simulink model "tilstandsmodelReducedOBS"  (Simulink 7.4)
settings: Solver=ode45  StartTime=0.0  StopTime=200  FixedStep=0.001  RelTol=1e-3
values from neighbouring files (symbols this model uses):
  A = [((-(Km^2)/(Rm*Jt))-(bs/Jt)) 0 0 0 ... (first row only)    [tilstandsREG.m]
  Aro = [0 ((3*g)/(lp*2));1 0]    [tilstandsREG.m]
  B = [1.292*(Km/(Jt*Rm)) ... (first row only)    [tilstandsREG.m]
  Bro = [1;0]    [tilstandsREG.m]
  C = [1 0 0 0 ... (first row only)    [tilstandsREG.m]
  Cro = [0 -(9*la*g)/(4*lp^2)]    [tilstandsREG.m]
  Dro = [-(3*la)/(2*lp)]    [tilstandsREG.m]
  F = Fe(:,1:4)    [tilstandsREG.m]
  Fi = Fe(:,5)    [tilstandsREG.m]
  Km = 0.022141706562986    (= 0.022141706563)    [pindregStart.m]    (also in tilstandsREG.m)
  Lro = (-place(Aro',Cro',[-35;-36]))'    [tilstandsREG.m]
  Rm = 0.807790757873553    (= 0.807790757874)    [pindregStart.m]    (also in tilstandsREG.m)
libraries: vrlib x3, simulink x1
settings Model: Creator=Skov  LastModifiedBy=Skov

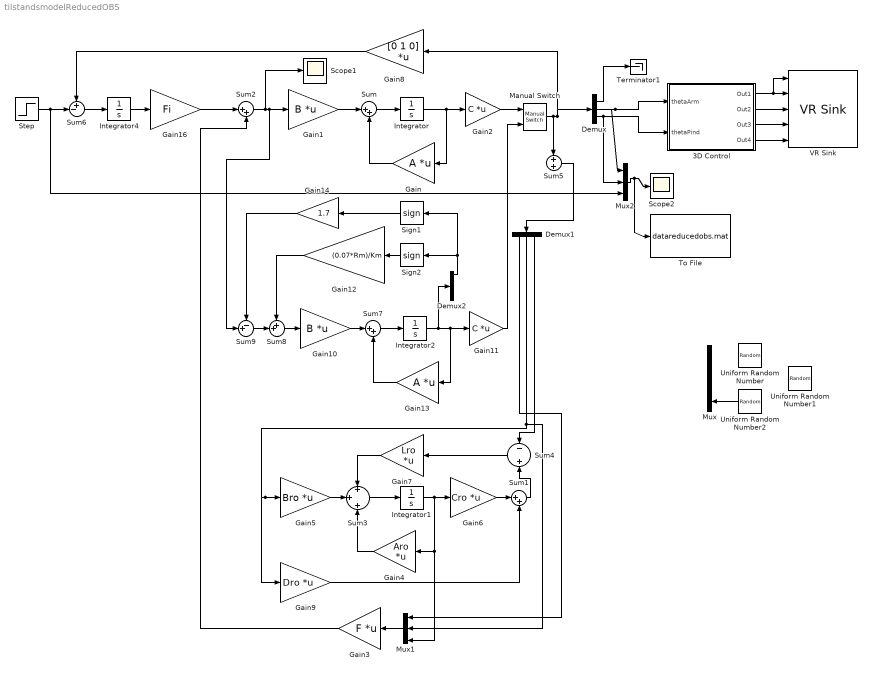
== system tilstandsmodelReducedOBS ==
  3D Control : Subsystem
  Demux : Demux  Outputs=3
  Demux1 : Demux  Outputs=3
  Demux2 : Demux
  Gain : Gain  Gain=A  Multiplication=Matrix(K*u)  ParameterDataType=fixdt(1, 16)  ParameterScaling=2^0  OutDataType=fixdt(1, 16)  OutScaling=2^0
  Gain1 : Gain  Gain=B  Multiplication=Matrix(K*u)  ParameterDataType=fixdt(1, 16)  ParameterScaling=2^0  OutDataType=fixdt(1, 16)  OutScaling=2^0
  Gain10 : Gain  Gain=B  Multiplication=Matrix(K*u)  ParameterDataType=fixdt(1, 16)  ParameterScaling=2^0  OutDataType=fixdt(1, 16)  OutScaling=2^0
  Gain11 : Gain  Gain=C  Multiplication=Matrix(K*u)  ParameterDataType=fixdt(1, 16)  ParameterScaling=2^0  OutDataType=fixdt(1, 16)  OutScaling=2^0
  Gain12 : Gain  Gain=(0.07*Rm)/Km  ParameterDataType=fixdt(1, 16)  ParameterScaling=2^0  OutDataType=fixdt(1, 16)  OutScaling=2^0
  Gain13 : Gain  Gain=A  Multiplication=Matrix(K*u)  ParameterDataType=fixdt(1, 16)  ParameterScaling=2^0  OutDataType=fixdt(1, 16)  OutScaling=2^0
  Gain14 : Gain  Gain=1.7  ParameterDataType=fixdt(1, 16)  ParameterScaling=2^0  OutDataType=fixdt(1, 16)  OutScaling=2^0
  Gain16 : Gain  Gain=Fi  ParameterDataType=fixdt(1, 16)  ParameterScaling=2^0  OutDataType=fixdt(1, 16)  OutScaling=2^0
  Gain2 : Gain  Gain=C  Multiplication=Matrix(K*u)  ParameterDataType=fixdt(1, 16)  ParameterScaling=2^0  OutDataType=fixdt(1, 16)  OutScaling=2^0
  Gain3 : Gain  Gain=F  Multiplication=Matrix(K*u)  ParameterDataType=fixdt(1, 16)  ParameterScaling=2^0  OutDataType=fixdt(1, 16)  OutScaling=2^0
  Gain4 : Gain  Gain=Aro  Multiplication=Matrix(K*u)  ParameterDataType=fixdt(1, 16)  ParameterScaling=2^0  OutDataType=fixdt(1, 16)  OutScaling=2^0
  Gain5 : Gain  Gain=Bro  Multiplication=Matrix(K*u)  ParameterDataType=fixdt(1, 16)  ParameterScaling=2^0  OutDataType=fixdt(1, 16)  OutScaling=2^0
  Gain6 : Gain  Gain=Cro  Multiplication=Matrix(K*u)  ParameterDataType=fixdt(1, 16)  ParameterScaling=2^0  OutDataType=fixdt(1, 16)  OutScaling=2^0
  Gain7 : Gain  Gain=Lro  Multiplication=Matrix(K*u)  ParameterDataType=fixdt(1, 16)  ParameterScaling=2^0  OutDataType=fixdt(1, 16)  OutScaling=2^0
  Gain8 : Gain  Gain=[0 1 0]  Multiplication=Matrix(K*u)  ParameterDataType=fixdt(1, 16)  ParameterScaling=2^0  OutDataType=fixdt(1, 16)  OutScaling=2^0
  Gain9 : Gain  Gain=Dro  Multiplication=Matrix(K*u)  ParameterDataType=fixdt(1, 16)  ParameterScaling=2^0  OutDataType=fixdt(1, 16)  OutScaling=2^0
  Integrator : Integrator  InitialCondition=[0 0 0 0]
  Integrator1 : Integrator  InitialCondition=[0 0]
  Integrator2 : Integrator  InitialCondition=[0 0 0 0]
  Integrator4 : Integrator  InitialCondition=[0]
  Manual Switch : simulink/Signal Routing/Manual Switch  SystemSampleTime=-1  sw=1  action=0  varsize=off
  Mux : Mux  Inputs=3
  Mux1 : Mux  Inputs=3
  Mux2 : Mux  Inputs=3
  Scope1 : Scope
      settings: YMin=-17.5  YMax=17.5
  Scope2 : Scope
      settings: YMin=-0.1  YMax=0.65
  Sign1 : Signum  SampleTime=0.01
  Sign2 : Signum  SampleTime=0.01
  Step : Step  After=pi/6  SampleTime=0
  Sum{,1..2,7} (4 alike) : Sum  Inputs=|++  OutDataType=fixdt(1, 16)  OutScaling=2^0
  Sum3 : Sum  Inputs=+|+|+  OutDataType=fixdt(1, 16)  OutScaling=2^0
  Sum4 : Sum  Inputs=-|+  OutDataType=fixdt(1, 16)  OutScaling=2^0
  Sum5 : Sum  Inputs=+|+  OutDataType=fixdt(1, 16)  OutScaling=2^0
  Sum6 : Sum  Inputs=+-|  OutDataType=fixdt(1, 16)  OutScaling=2^0
  Sum8 : Sum  Inputs=++|  OutDataType=fixdt(1, 16)  OutScaling=2^0
  Sum9 : Sum  Inputs=-+|  OutDataType=fixdt(1, 16)  OutScaling=2^0
  Terminator1 : Terminator
  To File : ToFile  Filename=datareducedobs.mat
  Uniform Random Number : UniformRandomNumber  Minimum=0  Seed=234567  SampleTime=0.1
  Uniform Random Number1 : UniformRandomNumber  Minimum=-pi/180  Maximum=pi/180  SampleTime=0.1
  Uniform Random Number2 : UniformRandomNumber  Minimum=-pi/180  Maximum=pi/180  SampleTime=0.1
  VR Sink : vrlib/VR Sink  InstantiateOnLoad=on  SampleTime=-1  ViewEnable=on  RemoteChange=off  RemoteView=on  FieldsWritten=Ball.rotation.4.1.double#Arm.rotation.4.1.double#Pind.translation.3.1.double#AP.translation.3.1.double#Pind.rotation.4.1.double  WorldFileName=VRML1.WRL  AutoView=off  VideoDimensions=[]
  wires:
  Integrator/1 -> Gain2/1, Gain/1
  Sum/1 -> Integrator/1
  Gain1/1 -> Sum/1
  Gain/1 -> Sum/2
  3D Control/1(Out1) -> VR Sink/1, VR Sink/2
  3D Control/2(Out2) -> VR Sink/3
  3D Control/3(Out3) -> VR Sink/4
  3D Control/4(Out4) -> VR Sink/5
  Demux/2 -> 3D Control/1(thetaArm), Mux2/1
  Demux/3 -> 3D Control/2(thetaPind), Mux2/2
  Integrator1/1 -> Gain6/1, Gain4/1, Mux1/3
  Sum3/1 -> Integrator1/1
  Gain4/1 -> Sum3/3
  Gain5/1 -> Sum3/2
  Sum4/1 -> Gain7/1
  Sum2/1 -> Scope1/1, Gain1/1, Sum9/2
  Gain7/1 -> Sum3/1
  Demux/1 -> Terminator1/1
  Gain8/1 -> Sum6/1
  Step/1 -> Sum6/2, Mux2/3
  Mux1/1 -> Gain3/1
  Gain6/1 -> Sum1/1
  Sum1/1 -> Sum4/2
  Gain9/1 -> Sum1/2
  Sum5/1 -> Demux1/1
  Demux1/2 -> Gain9/1, Gain5/1, Mux1/2
  Demux1/1 -> Mux1/1
  Demux1/3 -> Sum4/1
  Gain2/1 -> Manual Switch/1
  Manual Switch/1 -> Gain8/1, Demux/1, Sum5/1
  Gain10/1 -> Sum7/1
  Integrator2/1 -> Gain11/1, Gain13/1, Demux2/1
  Sum7/1 -> Integrator2/1
  Gain13/1 -> Sum7/2
  Sum8/1 -> Gain10/1
  Sign2/1 -> Gain12/1
  Demux2/1 -> Sign2/1, Sign1/1
  Gain12/1 -> Sum8/1
  Gain11/1 -> Manual Switch/2
  Mux2/1 -> Scope2/1, To File/1
  Sum9/1 -> Sum8/2
  Sign1/1 -> Gain14/1
  Uniform Random Number2/1 -> Mux/3
  Gain3/1 -> Sum2/2
  Gain16/1 -> Sum2/1
  Sum6/1 -> Integrator4/1
  Integrator4/1 -> Gain16/1
  Gain14/1 -> Sum9/1

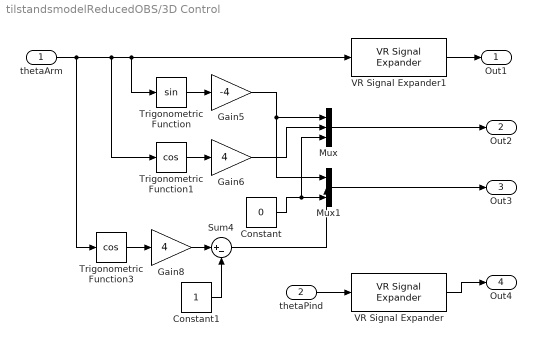
== system tilstandsmodelReducedOBS/3D Control ==
  thetaArm : Inport  OutDataType=fixdt(1, 16)  OutScaling=2^0
  thetaPind : Inport  Port=2  OutDataType=fixdt(1, 16)  OutScaling=2^0
  Constant : Constant  Value=0  OutDataType=fixdt(1, 16)  OutScaling=2^0
  Constant1 : Constant  OutDataType=fixdt(1, 16)  OutScaling=2^0
  Gain5 : Gain  Gain=-4  ParameterDataType=fixdt(1, 16)  ParameterScaling=2^0  OutDataType=fixdt(1, 16)  OutScaling=2^0
  Gain6 : Gain  Gain=4  ParameterDataType=fixdt(1, 16)  ParameterScaling=2^0  OutDataType=fixdt(1, 16)  OutScaling=2^0
  Gain8 : Gain  Gain=4  ParameterDataType=fixdt(1, 16)  ParameterScaling=2^0  OutDataType=fixdt(1, 16)  OutScaling=2^0
  Mux : Mux  Inputs=3
  Mux1 : Mux  Inputs=3
  Sum4 : Sum  Inputs=|+-  OutDataType=fixdt(1, 16)  OutScaling=2^0
  Trigonometric Function : Trigonometry
  Trigonometric Function1 : Trigonometry  Operator=cos
  Trigonometric Function3 : Trigonometry  Operator=cos
  VR Signal Expander : vrlib/VR Signal Expander  SystemSampleTime=-1  outwidth=4  outidx=[4]
  VR Signal Expander1 : vrlib/VR Signal Expander  SystemSampleTime=-1  outwidth=4  outidx=[4]
  Out1 : Outport  OutDataType=fixdt(1, 16)  OutScaling=2^0
  Out2 : Outport  Port=2  OutDataType=fixdt(1, 16)  OutScaling=2^0
  Out3 : Outport  Port=3  OutDataType=fixdt(1, 16)  OutScaling=2^0
  Out4 : Outport  Port=4  OutDataType=fixdt(1, 16)  OutScaling=2^0
  wires:
  Trigonometric Function/1 -> Gain5/1
  Gain5/1 -> Mux/1, Mux1/1
  Trigonometric Function1/1 -> Gain6/1
  Gain6/1 -> Mux/2
  Constant/1 -> Mux/3, Mux1/3
  Mux/1 -> Out2/1
  Trigonometric Function3/1 -> Gain8/1
  Gain8/1 -> Sum4/1
  Constant1/1 -> Sum4/2
  Sum4/1 -> Mux1/2
  Mux1/1 -> Out3/1
  thetaArm/1 -> Trigonometric Function1/1, Trigonometric Function/1, VR Signal Expander1/1, Trigonometric Function3/1
  thetaPind/1 -> VR Signal Expander/1
  VR Signal Expander/1 -> Out4/1
  VR Signal Expander1/1 -> Out1/1
